simulink model "RefSub"  (R2026a)
settings: configuration reference "testConfig" (kept outside this file)
model workspace (MAT data in the model file):
  p1 = Simulink.Parameter
  p1.Value = [1  2; 3  4]
  p1.Complexity = 'real'
  p1.Dimensions = [2 2]
  p1.DataType = 'int8'
  ps = Simulink.Parameter
  ps.Value.p1 = 1
  ps.Value.psi.psi1 = 1
  ps.Complexity = 'real'
  ps.Dimensions = [1 1]
  ps.DataType = 'struct'
settings Model: DataDictionary=MyParams.sldd  ParameterArgumentNames=p1,ps  Creator=tomha  LastModifiedBy=toma
settings ConfigSetRef: SourceName=testConfig

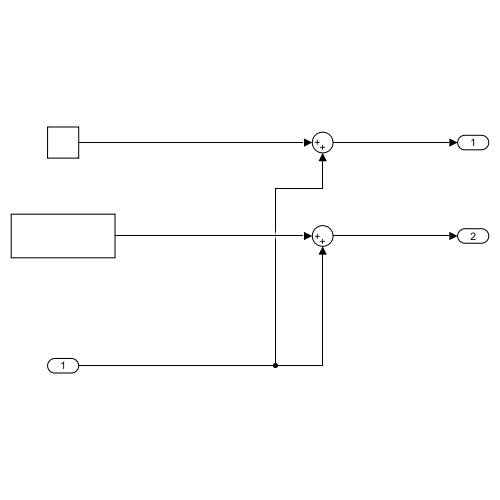
[thumbnail: Simulink's stored preview of the top-level diagram]
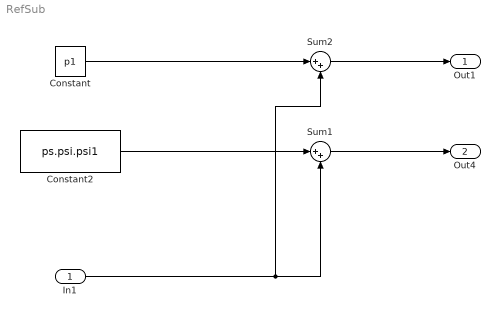
== system RefSub ==
  In1 : Inport  OutDataTypeStr=double  PortDimensions=1  SampleTime=[0.20000000000000001,0]
  Constant : Constant  Value=p1
  Constant2 : Constant  Value=ps.psi.psi1
  Sum1 : Sum  Inputs=|++
  Sum2 : Sum  Inputs=|++
  Out1 : Outport  OutDataTypeStr=double  PortDimensions=[2 2]  SampleTime=[0.20000000000000001,0]
  Out4 : Outport  Port=2  OutDataTypeStr=double  PortDimensions=1  SampleTime=[0.20000000000000001,0]
  wires:
  Constant2/1 -> Sum1/1
  Sum1/1 -> Out4/1
  Constant/1 -> Sum2/1
  Sum2/1 -> Out1/1
  In1/1 -> Sum2/2, Sum1/2
